simulink model "FM"  (R2020b)
settings: Solver=VariableStepAuto  StartTime=0.0  StopTime=10.0  RelTol=1e-3
libraries: commsynccomp2 x1, dsparch4 x1, dspsigops x1
settings Model: Creator=taone  LastModifiedBy=htn
settings SFSimCC: CustomCodeUndefinedFunction=UseInterfaceOnly

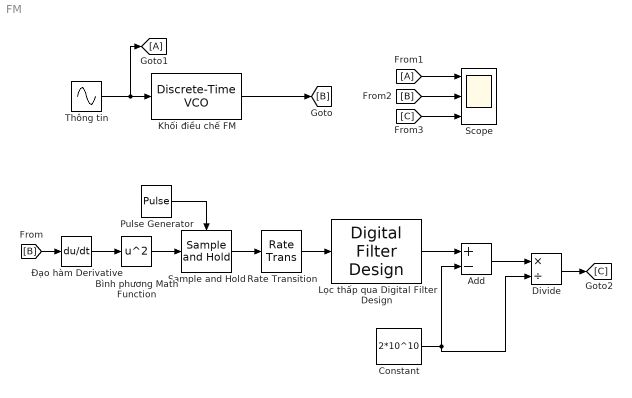
== system FM ==
  Add : Sum  Inputs=+-
  Bình phương Math Function : Math  Operator=square  SignedPower=on  SaturateOnIntegerOverflow=on
  Constant : Constant  Value=2*10^10
  Divide : Product  Inputs=*/
  "Khối điều chế FM " : commsynccomp2/Discrete-Time VCO  Ac=5  Fc=5000  Kc=1500  Ph=0  ts=1/30000
      settings: SourceProductBaseCode=CM
  Lọc thấp qua Digital Filter Design : dsparch4/Digital Filter Design  mwdsp_browser_bugfix_var=off
  Pulse Generator : DiscretePulseGenerator  PulseType=Time based  Period=1/30000  PulseWidth=50
  Rate Transition : RateTransition  OutPortSampleTime=1/30000
  Sample and Hold : dspsigops/Sample and Hold  trig=Rising edge  initCond=0  latchinput=off
  Scope : Scope  NumInputPorts=3
  "Thông tin " : Sin  Amplitude=2  Frequency=2*pi*500  SampleTime=1/30000
  Đạo hàm Derivative : Derivative
  wires:
  Add/1 -> Divide/1
  "Thông tin "/1 -> "Khối điều chế FM "/1, [A]
  Bình phương Math Function/1 -> Sample and Hold/1
  [C] -> Scope/3
  Rate Transition/1 -> Lọc thấp qua Digital Filter Design/1
  Lọc thấp qua Digital Filter Design/1 -> Add/1
  "Khối điều chế FM "/1 -> [B]
  [B] -> Scope/2
  Sample and Hold/1 -> Rate Transition/1
  [B] -> Đạo hàm Derivative/1
  Divide/1 -> [C]
  Pulse Generator/1 -> Sample and Hold/Trigger
  Constant/1 -> Divide/2, Add/2
  Đạo hàm Derivative/1 -> Bình phương Math Function/1
  [A] -> Scope/1
